simulink model "gnc"  (R2025b)
settings: Solver=ode2  StartTime=0.0  StopTime=inf  FixedStep=1/100  RelTol=1e-3
PreLoadFcn:
  | gnc_PreLoadFcn
undefined symbols (not defined in the file or in its folder): DiscIntNeverNeededParam, dspblkCoreblockFVToolHelper, gcbh
libraries: simulink_extras x7, simulink x5, eeGeneralControl x5
(part 4 of 4)

== matlab function gnc/Modal/MATLAB Function6 ==
  data: axis_modes input; xLat output size=4; gachi_m input; chi output; xLon output; rates input; Vk input; attitude input
function [xLat,chi,xLon] = fcn(axis_modes,gachi_m,rates,Vk,attitude)
%#codegen

if norm(Vk)>1
    chi = gachi_m(2);
    gamma = gachi_m(1);
else
    chi = attitude(4); % psi
    gamma = single(0);
end

if axis_modes(3) == int8(20) %LNAV_ALGN: PSI --> ZETA
    xLat = [rates(3); rates(1); attitude(5); attitude(4)]; %psi
else
    xLat = [rates(3); rates(1); attitude(5); attitude(3)]; %beta
end

if axis_modes(2) == int8(21) %VNAV_THETA: THETA --> ETA
    xLon = [attitude(2); rates(2); Vk; gamma]; %theta
else
    xLon = [attitude(1); rates(2); Vk; gamma]; %alpha
end

== matlab function gnc/INDI/Rates to surfaces&brakes/Incremental_inversion/rad2cmd ==
  data: act_limits input; u input single size=3; y output single size=3
function y = fcn(act_limits,u)

y = u./(act_limits*pi/180); %scale control surface commands to [-1,1]

== matlab function gnc/Mixer/MATLAB Function2 ==
  data: params input Bus: gnc_parameterBus; controls_in input single size=4; controls_out output single size=8; ap_mode input
function controls_out = fcn(params,controls_in,ap_mode)
controls_out = zeros(8,1,'single');

controls_out(1) = controls_in(1);

% ail = controls_in(2)*2/sqrt(2);%45° deflection
% ele = controls_in(3)*2/sqrt(2);%45° deflection
% rud = controls_in(4)*2/sqrt(2);%45° deflection
ail = controls_in(2)*2/3;
ele = controls_in(3)*2/3;
rud = controls_in(4)*2/3;

ail_rud = ail;% + rud;

ail_rud_min = max(-ele-1,ele-1);
ail_rud_max = min(-ele+1,ele+1);
ail_rud_ltd = min(max(ail_rud,ail_rud_min),ail_rud_max);

if ap_mode <= 1
    if params.trim_ail_prio %ail
        ele = single(0);
    else %ele
        ail_rud_ltd = single(0);
    end
end

controls_out(5) = ele + ail_rud_ltd;
controls_out(6) = ele - ail_rud_ltd;

== matlab function gnc/INDI/MATLAB Function1 ==
  data: Vk input single; q_dyn output single; gncConsts parameter Bus: gnc_constantsBus
function q_dyn = fcn(Vk,gncConsts)

Vk = max(Vk,single(10));
q_dyn    = 0.5*gncConsts.rho*Vk^2;

== matlab function gnc/INDI/Rates to surfaces&brakes/Diff and Filter IMU/fromRPAS/MATLAB Function ==
  data: diff_num output single; diff_den output single; omega input single; zeta input single; filt_num output single; filt_den output single
function [diff_num,diff_den,filt_num,filt_den]  = tbv(omega, zeta)

T = single(0.01);
w = omega;
z = zeta;

scale = T^2*w^2+4*T*w*z+4;

diff_num = [2*T*w^2 0 -2*T*w^2]/scale;
diff_den = [T^2*w^2+4*T*w*z+4 2*T^2*w^2-8 T^2*w^2-4*T*w*z+4]/scale;

filt_num = [T^2*w^2, 2*T^2*w^2, T^2*w^2]/scale;
filt_den = [T^2*w^2+4*T*w*z+4 2*T^2*w^2-8 T^2*w^2-4*T*w*z+4]/scale;

== matlab function gnc/Mixer/PWM Limiter ==
  data: parameter input; controls input; controlsLtd output single
function controlsLtd = fcn(parameter,controls)

% limUp = [parameter.rc.max1,parameter.rc.max2,parameter.rc.max3,parameter.rc.max4,parameter.rc.max5,parameter.rc.max6,parameter.rc.max7,parameter.rc.max8,parameter.rc.max9,parameter.rc.max10,parameter.rc.max11,parameter.rc.max12,parameter.rc.max13,parameter.rc.max14,parameter.rc.max15,parameter.rc.max16];
% limDown = [parameter.rc.min1,parameter.rc.min2,parameter.rc.min3,parameter.rc.min4,parameter.rc.min5,parameter.rc.min6,parameter.rc.min7,parameter.rc.min8,parameter.rc.min9,parameter.rc.min10,parameter.rc.min11,parameter.rc.min12,parameter.rc.min13,parameter.rc.min14,parameter.rc.min15,parameter.rc.min16];
% trim = [parameter.rc.trim1,parameter.rc.trim2,parameter.rc.trim3,parameter.rc.trim4,parameter.rc.trim5,parameter.rc.trim6,parameter.rc.trim7,parameter.rc.trim8,parameter.rc.trim9,parameter.rc.trim10,parameter.rc.trim11,parameter.rc.trim12,parameter.rc.trim13,parameter.rc.trim14,parameter.rc.trim15,parameter.rc.trim16];
% 
% controlsLtd = zeros(size(controls));
% 
% if parameter.rc.rcType == 2
%     center = 1500;
%     range = 400;
% else
%     center = 1514;
%     range = 420;
% end
% 
% for i=1:length(controls)
%     if controls(i)>0
%         controlsLtd(i) = controls(i)*(limUp(i)-trim(i))/range+(trim(i)-center)/range;
%     else
%         controlsLtd(i) = controls(i)*(trim(i)-limDown(i))/range+(trim(i)-center)/range;
%     end
% end

controlsLtd = single(controls);

== matlab function gnc/Subsystem2/Actuator_Model/Subsystem1/MATLAB Function ==
  data: u input; y output uint8
function y = fcn(u)
% assign rc-modes depending on the switch position
if u < single(-0.33) %test_controls
    y = uint8(1);
elseif u < single(0.33) %steady_state
    y = uint8(2);
else %wp_tracking
    y = uint8(3);
end

== matlab function gnc/Subsystem2/Actuator_Model/Actuator Model/MATLAB Function1 ==
  data: in input; out output
function out = fcn(in)

out = [in(1:3);0.5*in(4)+0.5]; %scale thrust from [-1,1] to [0,1]

== matlab function gnc/Subsystem2/Actuator_Model/Actuator Model/cmd2deg ==
  data: act_limits input single; u input single; y output single
function y = fcn(act_limits,u)

y = u.*(act_limits*pi/180);

== matlab function gnc/Mixer/revert_alloc ==
  data: in input; out output
function out = fcn(in)
out = zeros(4,1);

out(1) = in(1); %thr
out(2) = 3/2*(in(5)-in(6))/2; %ail
out(3) = 3/2*(in(5)+in(6))/2; %ele
out(4) = 0; %rud

== matlab function gnc/Subsystem2/acc transformation4 ==
  data: acc_b input; euler input; acc_g output
function acc_g  = acc_transform(acc_b,euler)
g=9.81;

tf3 = [cos(-euler(3)) sin(-euler(3)) 0; -sin(-euler(3)) cos(-euler(3)) 0; 0 0 1];
tf2 = [cos(-euler(2)) 0 -sin(-euler(2)); 0 1 0; sin(-euler(2)) 0 cos(-euler(2))];
tf1 = [1 0 0; 0 cos(-euler(1)) sin(-euler(1)); 0 -sin(-euler(1)) cos(-euler(1))];

acc_g = tf3*tf2*tf1*(acc_b)+[0;0;g];

% T1 = [1 0 0; 0 cos(-eul(1)) sin(-eul(1)); 0 -sin(-eul(1)) cos(-eul(1))];
% T2 = [cos(-eul(2)) 0 -sin(-eul(2)); 0 1 0; sin(-eul(2)) 0 cos(-eul(2))];
% acc_g=T2*T1*acc_b;% + cross(-rates,(T2*T1)\vel);
% acc_g = acc_g + [0;0;g];

== matlab function gnc/Subsystem2/Actuator_Model/Actuator Model/limit control output ==
  data: u input single; y output single
function y = control_output_sat(u)

y = zeros(size(u),'single');
y(:) = min(max(u(:),-1),1);

end

== matlab function gnc/Subsystem2/Actuator_Model/Actuator Model/limit control output3 ==
  data: u input single; y output single
function y = control_output_sat(u)

y = zeros(size(u),'single');
y(:) = min(max(u(:),0),1);

end

== matlab function gnc/Subsystem2/Angles Estimation ==
  data: speeds output single size=2; euler input single size=3; vel input single size=3; Va input; track output single size=2
function [speeds,track] = anglesEstimation(euler,vel,Va)

Vk = norm(vel);
if isnan(Va) || Va < single(2)
    Va = single(2);
end
if isnan(Vk)
    Vk = single(0);
end

if Vk > 2
    chi = atan2(vel(2), vel(1));
    gamma = asin(-vel(3)/norm(vel));
    V_A   = Va;
else
    chi = euler(3); % psi
    gamma = single(0); %attitude(2); %theta
    V_A   = Vk;
end

% if param.VaDisabled
%     V_A   = Vk;
% end

track = [gamma, chi]';
speeds = [Vk, V_A]';
end

== matlab function gnc/Subsystem2/MATLAB Function ==
  data: quat input; eul_rad output
function eul_rad=quat2euler(quat)

eul_rad = single([0;0;0]);
ysqr = quat(3) * quat(3);

t0 = 2 * (quat(1) * quat(2) + quat(3) * quat(4));
t1 = 1 - 2 * (quat(2) * quat(2) + ysqr);
eul_rad(1) = atan2(t0, t1);

t2 = 2 * (quat(1) * quat(3) - quat(4) * quat(2));
if t2 > 1
    t2 = single(1);
elseif t2 < -1
    t2 = -single(1);
end
eul_rad(2) = asin(t2);

t3 = 2 * (quat(1) * quat(4) + quat(2) * quat(3));
t4 = 1 - 2 * (ysqr + quat(4) * quat(4));
eul_rad(3) = atan2(t3, t4);

end

== matlab function gnc/Subsystem2/Subsystem/MATLAB Function ==
  data: acc_k input; gachi_dot output single size=2; Vk input
function gachi_dot = fcn(acc_k,Vk)
if Vk < single(0.5)
    Vk = single(0.5);
end

gachi_dot = [-acc_k(3);acc_k(2)]/Vk;

== matlab function gnc/Subsystem2/Subsystem/exception_handler ==
  data: u input single; y output single
function y = fcn(u)

if u>=1 && u<=6
    y=u;
else
    y=single(1);
end

== matlab function gnc/Subsystem2/Subsystem2/exception_handler ==
  data: u input single; y output single
function y = fcn(u)

if u>=1 && u<=6
    y=u;
else
    y=single(1);
end

== matlab function gnc/Mixer/scale_thr ==
  data: in input single size=4; out output single size=4
function out = fcn(in)

out = in;
out(4) = 2*in(4)-1; %scale thrust from [0,1] to [-1,1]

== matlab function gnc/Subsystem2/acc transformation ==
  data: gachi_m input; acc_g input; acc_k output
function acc_k  = acc_transform(gachi_m,acc_g)

tf2 = [cos(gachi_m(1)) 0 -sin(gachi_m(1)); 0 1 0; sin(gachi_m(1)) 0 cos(gachi_m(1))];
tf3 = [cos(gachi_m(2)) sin(gachi_m(2)) 0; -sin(gachi_m(2)) cos(gachi_m(2)) 0; 0 0 1];

acc_k = tf2*tf3*(acc_g);

== matlab function gnc/INDI/Rates to surfaces&brakes/Diff and Filter IMU/fromRPAS/Subsystem/MATLAB Function ==
  data: omega input single; zeta input single; filt_num output single; filt_den output single
function [filt_num,filt_den]  = tbv(omega, zeta)

T = single(0.01);
w = omega;
z = zeta;

scale = T^2*w^2+4*T*w*z+4;

filt_num = [T^2*w^2, 2*T^2*w^2, T^2*w^2]/scale;
filt_den = [T^2*w^2+4*T*w*z+4 2*T^2*w^2-8 T^2*w^2-4*T*w*z+4]/scale;

== matlab function gnc/Guidance/ATOL_Guidance ==
  settings: updateMethod=DISCRETE
  data: AP_mode input uint8; params input Bus: gnc_parameterBus; guidance_out output Bus: guidance_cmd; cruise_guid input single size=3
function guidance_out  = Guidance(AP_mode,params,cruise_guid)

%% Instantiate output signals
thetaCmd = single(0);
psiCmd   = single(0);
phiCmd   = single(0);
gammaCmd  = single(0);
chiCmd   = single(0);
vCmd      = single(0);

%% Guidance
switch AP_mode
    case 1 % Test controls on ground
        phiCmd = single(0);
        thetaCmd = single(0);
        psiCmd = single(0);
    case 2 %track following
        gammaCmd = params.guidance.gamma_cmd*pi/180;
        phiCmd = single(0); %wings level
        vCmd = params.guidance.v_cmd;
    case 3
        if params.wp_tracking==1 %enter cruise
            vCmd = cruise_guid(3);
            gammaCmd = cruise_guid(1);
            chiCmd = cruise_guid(2);
        else
            vCmd = params.guidance.v_cmd;
            gammaCmd = params.guidance.gamma_cmd*pi/180;
            chiCmd = params.guidance.chi_cmd*pi/180;
        end
end

% Limit pitch and yaw/chi
chiCmd = mod((chiCmd+pi),2*pi)-pi;
psiCmd = mod((psiCmd+pi),2*pi)-pi;

% Summarize command values
guidance_out.roll_lim = single(45*pi/180);
guidance_out.act_cmd = zeros(6,1,'single');
guidance_out.rte_cmd = zeros(3,1,'single');
guidance_out.att_cmd = [single(0);thetaCmd;single(0);psiCmd;phiCmd];
guidance_out.trk_cmd = [gammaCmd;chiCmd;vCmd];

end

== matlab function gnc/Subsystem2/MATLAB Function2 ==
  data: param input Bus: gnc_parameterBus; acc_raw input Bus: sensor_accel_bus; aero_est output; acc_filt input; acc_b output
function [aero_est,acc_b] = fcn(param,acc_raw,acc_filt)
pix_orientation = [param.nav.pix_roll;param.nav.pix_pitch;param.nav.pix_yaw];

T1 = [1 0 0;0 cos(pix_orientation(1)) sin(pix_orientation(1));0 -sin(pix_orientation(1)) cos(pix_orientation(1))];
T2 = [cos(pix_orientation(2)) 0 -sin(pix_orientation(2));0 1 0;sin(pix_orientation(2)) 0 cos(pix_orientation(2))];
T3 = [cos(pix_orientation(3)) sin(pix_orientation(3)) 0;-sin(pix_orientation(3)) cos(pix_orientation(3)) 0;0 0 1];
T = T1*T2*T3;

if isequal(param.imu_filt_ang_acc,single(1))
    acc_b = acc_filt;
else
    acc_b = T*[acc_raw.x;acc_raw.y;acc_raw.z];
end

aero_est = [(acc_b(3)+9.80884)/-155.1208;acc_b(2)/-9.0732];

== matlab function gnc/Mixer/MATLAB Function1 ==
  data: params input Bus: gnc_parameterBus; controls output single size=4; ap_controls input single size=4; rc_controls input single
function controls = fcn(params,ap_controls,rc_controls)
com_authority = [params.authority.chan1,params.authority.chan2,params.authority.chan3,params.authority.chan4];

controls = zeros(4,1,'single');

switch params.trim_switch
    case 1 %trim mode active
        controls(1:4) = rc_controls(1:4);
    case 2
        for i = 1:length(com_authority)
            controls(i) = (1-com_authority(i))*rc_controls(i) + com_authority(i)*ap_controls(i);
        end
    otherwise
        controls(1:4) = ap_controls(1:4);
end

== matlab function gnc/INDI/Rates to surfaces&brakes/Diff and Filter IMU/fromRPAS/Subsystem/MATLAB Function1 ==
  data: omega input single; zeta input single; filt_num output single; filt_den output single
function [filt_num,filt_den]  = tbv(omega, zeta)

T = single(0.01);
w = omega;
z = zeta;

scale = T^2*w^2+4*T*w*z+4;

filt_num = [T^2*w^2, 2*T^2*w^2, T^2*w^2]/scale;
filt_den = [T^2*w^2+4*T*w*z+4 2*T^2*w^2-8 T^2*w^2-4*T*w*z+4]/scale;

== matlab function gnc/INDI/Rates to surfaces&brakes/Diff and Filter IMU/fromRPAS/Subsystem/MATLAB Function2 ==
  data: omega input single; zeta input single; filt_num output single; filt_den output single
function [filt_num,filt_den]  = tbv(omega, zeta)

T = single(0.01);
w = omega;
z = zeta;

scale = T^2*w^2+4*T*w*z+4;

filt_num = [T^2*w^2, 2*T^2*w^2, T^2*w^2]/scale;
filt_den = [T^2*w^2+4*T*w*z+4 2*T^2*w^2-8 T^2*w^2-4*T*w*z+4]/scale;

== matlab function gnc/INDI/Rates to surfaces&brakes/Diff and Filter IMU/fromRPAS/Subsystem/MATLAB Function3 ==
  data: omega input single; zeta input single; filt_num output single; filt_den output single
function [filt_num,filt_den]  = tbv(omega, zeta)

T = single(0.01);
w = omega;
z = zeta;

scale = T^2*w^2+4*T*w*z+4;

filt_num = [T^2*w^2, 2*T^2*w^2, T^2*w^2]/scale;
filt_den = [T^2*w^2+4*T*w*z+4 2*T^2*w^2-8 T^2*w^2-4*T*w*z+4]/scale;

== matlab function gnc/INDI/Rates to surfaces&brakes/Diff and Filter IMU/fromRPAS/Subsystem/MATLAB Function4 ==
  data: omega input single; zeta input single; filt_num output single; filt_den output single
function [filt_num,filt_den]  = tbv(omega, zeta)

T = single(0.01);
w = omega;
z = zeta;

scale = T^2*w^2+4*T*w*z+4;

filt_num = [T^2*w^2, 2*T^2*w^2, T^2*w^2]/scale;
filt_den = [T^2*w^2+4*T*w*z+4 2*T^2*w^2-8 T^2*w^2-4*T*w*z+4]/scale;

== matlab function gnc/INDI/Rates to surfaces&brakes/Diff and Filter IMU/fromRPAS/Subsystem/MATLAB Function5 ==
  data: omega input single; zeta input single; filt_num output single; filt_den output single
function [filt_num,filt_den]  = tbv(omega, zeta)

T = single(0.01);
w = omega;
z = zeta;

scale = T^2*w^2+4*T*w*z+4;

filt_num = [T^2*w^2, 2*T^2*w^2, T^2*w^2]/scale;
filt_den = [T^2*w^2+4*T*w*z+4 2*T^2*w^2-8 T^2*w^2-4*T*w*z+4]/scale;

== matlab function gnc/INDI/Rates to surfaces&brakes/Diff and Filter IMU/fromRPAS/Subsystem/MATLAB Function10 ==
  data: omega input single; zeta input single; filt_num output single; filt_den output single
function [filt_num,filt_den]  = tbv(omega, zeta)

T = single(0.01);
w = omega;
z = zeta;

scale = T^2*w^2+4*T*w*z+4;

filt_num = [T^2*w^2, 2*T^2*w^2, T^2*w^2]/scale;
filt_den = [T^2*w^2+4*T*w*z+4 2*T^2*w^2-8 T^2*w^2-4*T*w*z+4]/scale;

== matlab function gnc/INDI/Rates to surfaces&brakes/Diff and Filter IMU/fromRPAS/Subsystem/MATLAB Function11 ==
  data: omega input single; zeta input single; filt_num output single; filt_den output single
function [filt_num,filt_den]  = tbv(omega, zeta)

T = single(0.01);
w = omega;
z = zeta;

scale = T^2*w^2+4*T*w*z+4;

filt_num = [T^2*w^2, 2*T^2*w^2, T^2*w^2]/scale;
filt_den = [T^2*w^2+4*T*w*z+4 2*T^2*w^2-8 T^2*w^2-4*T*w*z+4]/scale;

== matlab function gnc/INDI/Rates to surfaces&brakes/Diff and Filter IMU/fromRPAS/Subsystem/MATLAB Function6 ==
  data: omega input single; zeta input single; filt_num output single; filt_den output single
function [filt_num,filt_den]  = tbv(omega, zeta)

T = single(0.01);
w = omega;
z = zeta;

scale = T^2*w^2+4*T*w*z+4;

filt_num = [T^2*w^2, 2*T^2*w^2, T^2*w^2]/scale;
filt_den = [T^2*w^2+4*T*w*z+4 2*T^2*w^2-8 T^2*w^2-4*T*w*z+4]/scale;

== matlab function gnc/INDI/Rates to surfaces&brakes/Diff and Filter IMU/fromRPAS/Subsystem/MATLAB Function7 ==
  data: omega input single; zeta input single; filt_num output single; filt_den output single
function [filt_num,filt_den]  = tbv(omega, zeta)

T = single(0.01);
w = omega;
z = zeta;

scale = T^2*w^2+4*T*w*z+4;

filt_num = [T^2*w^2, 2*T^2*w^2, T^2*w^2]/scale;
filt_den = [T^2*w^2+4*T*w*z+4 2*T^2*w^2-8 T^2*w^2-4*T*w*z+4]/scale;

== matlab function gnc/INDI/Rates to surfaces&brakes/Diff and Filter IMU/fromRPAS/Subsystem/MATLAB Function8 ==
  data: omega input single; zeta input single; filt_num output single; filt_den output single
function [filt_num,filt_den]  = tbv(omega, zeta)

T = single(0.01);
w = omega;
z = zeta;

scale = T^2*w^2+4*T*w*z+4;

filt_num = [T^2*w^2, 2*T^2*w^2, T^2*w^2]/scale;
filt_den = [T^2*w^2+4*T*w*z+4 2*T^2*w^2-8 T^2*w^2-4*T*w*z+4]/scale;

== matlab function gnc/INDI/Rates to surfaces&brakes/Diff and Filter IMU/fromRPAS/Subsystem/MATLAB Function9 ==
  data: omega input single; zeta input single; filt_num output single; filt_den output single
function [filt_num,filt_den]  = tbv(omega, zeta)

T = single(0.01);
w = omega;
z = zeta;

scale = T^2*w^2+4*T*w*z+4;

filt_num = [T^2*w^2, 2*T^2*w^2, T^2*w^2]/scale;
filt_den = [T^2*w^2+4*T*w*z+4 2*T^2*w^2-8 T^2*w^2-4*T*w*z+4]/scale;

== matlab function gnc/Modal/limit control output ==
  data: u input; y output single
function y = control_output_sat(u)

y = zeros(size(u),'single');
y(:) = min(max(u(:),-1),1);

end

== matlab function gnc/MATLAB Function ==
  data: ref_lla input; asl input; agl output
function agl = fcn(ref_lla,asl)

agl = asl+ref_lla(3)*1e-3; %down positive
